simulink model "generic_HELP_ME_mu"  (R2025a)
settings: Solver=ode45  StartTime=0.0  StopTime=12  RelTol=1e-3  EnableMultiTasking=on
values from neighbouring files (symbols this model uses):
  Battery =     [Battery_A123_Pack_204s2p_Final.mat]
  cs_tyre = 2.0e5    (= 200000)    [mu_estimator_parameters.m]
  dOCV_dSoC = gradient(OCV, SoC_bp)    [SoCOcv.m]
  dR0 = gradient(R0, SoC_L)    [SoCOcv.m]
  eps_vx = 0.5    [mu_estimator_parameters.m]
  fz_max = 6000    [mu_estimator_parameters.m]
  fz_min = 300    [mu_estimator_parameters.m]
  h_cg = 0.55    [mu_estimator_parameters.m]
  lf = 1.214    [mu_estimator_parameters.m]
  lr = 1.505    [mu_estimator_parameters.m]
  r0 = 0.344    [mu_estimator_parameters.m]
  re_max = 0.33    [mu_estimator_parameters.m]
  re_min = 0.28    [mu_estimator_parameters.m]
  SoC_bp = Table_SoCvsOCV.LUT.SoC_percent    [SoCOcv.m]
  SoC_L = Battery.SOC_LUT    [SoCOcv.m]
  Table_SoCvsOCV = load("SoC_to_Voltage_LUT_10000-GON.mat")    [SoCOcv.m]
  tw_f = 1.571    [mu_estimator_parameters.m]
  tw_r = 1.581    [mu_estimator_parameters.m]
undefined symbols (not defined in the file or in its folder): DiscIntNeverNeededParam, Init_SoC
libraries: CarMaker4SL x61, simulink x1
(part 4 of 4)

== matlab function generic_HELP_ME_mu/CarMaker/MATLAB Function28 ==
  data: mhat input; fz_fl output; ax_eff input; ay input; lf input; lr input; h_cg input; fz_fr output; fz_rl output; fz_rr output; tw_f input; tw_r input; fz_front_total output; fz_rear_total output
function [fz_fl, fz_fr, fz_rl, fz_rr, fz_front_total, fz_rear_total] = ...
    vertical_load_combined(mhat, ax_eff, ay, lf, lr, h_cg, tw_f, tw_r)

g = 9.81;
kf = 0.55;
kr = 0.45;
fz_min = 300;

L = lf + lr;

% Transfert longitudinal
fz_front_total = (mhat * g * lr - mhat * ax_eff * h_cg) / L;
fz_rear_total  = (mhat * g * lf + mhat * ax_eff * h_cg) / L;

% Transfert lateral
dfz_f_lat = (mhat * ay * h_cg / tw_f) * kf;
dfz_r_lat = (mhat * ay * h_cg / tw_r) * kr;

% Charges roue par roue
fz_fl = fz_front_total/2 + dfz_f_lat/2;
fz_fr = fz_front_total/2 - dfz_f_lat/2;

fz_rl = fz_rear_total/2 + dfz_r_lat/2;
fz_rr = fz_rear_total/2 - dfz_r_lat/2;

% Saturation mini
fz_fl = max(fz_fl, fz_min);
fz_fr = max(fz_fr, fz_min);
fz_rl = max(fz_rl, fz_min);
fz_rr = max(fz_rr, fz_min);

% Totaux recalcules
fz_front_total = fz_fl + fz_fr;
fz_rear_total  = fz_rl + fz_rr;

== matlab function generic_HELP_ME_mu/CarMaker/MATLAB Function29 ==
  data: fz_fl input; re_fl output; fz_fr input; fz_rl input; fz_rr input; re_fr output; re_rl output; re_rr output; r0 input; cs_tyre input; re_min input; re_max input
function [re_fl, re_fr, re_rl, re_rr] = ...
    effective_radius(fz_fl, fz_fr, fz_rl, fz_rr, r0, cs_tyre, re_min, re_max)

re_fl = r0 - (2/3) * (fz_fl / cs_tyre);
re_fr = r0 - (2/3) * (fz_fr / cs_tyre);
re_rl = r0 - (2/3) * (fz_rl / cs_tyre);
re_rr = r0 - (2/3) * (fz_rr / cs_tyre);

re_fl = min(max(re_fl, re_min), re_max);
re_fr = min(max(re_fr, re_min), re_max);
re_rl = min(max(re_rl, re_min), re_max);
re_rr = min(max(re_rr, re_min), re_max);

== matlab function generic_HELP_ME_mu/CarMaker/MATLAB Function30 ==
  data: vx input; slip_fl output; omega_fl input; omega_fr input; omega_rl input; slip_fr output; slip_rl output; slip_rr output; omega_rr input; re_fl input; re_fr input; re_rl input; re_rr input; eps_vx input
function [slip_fl, slip_fr, slip_rl, slip_rr] = ...
    slip_estimator(vx, omega_fl, omega_fr, omega_rl, omega_rr, ...
                        re_fl, re_fr, re_rl, re_rr, eps_vx)

if abs(vx) < eps_vx
    slip_fl = 0;
    slip_fr = 0;
    slip_rl = 0;
    slip_rr = 0;
else
    slip_fl = (vx - omega_fl * re_fl) / max(abs(vx), eps_vx);
    slip_fr = (vx - omega_fr * re_fr) / max(abs(vx), eps_vx);
    slip_rl = (vx - omega_rl * re_rl) / max(abs(vx), eps_vx);
    slip_rr = (vx - omega_rr * re_rr) / max(abs(vx), eps_vx);

    slip_fl = min(max(slip_fl, 0), 1);
    slip_fr = min(max(slip_fr, 0), 1);
    slip_rl = min(max(slip_rl, 0), 1);
    slip_rr = min(max(slip_rr, 0), 1);
end

== matlab function generic_HELP_ME_mu/CarMaker/EKF ==
  settings: updateMethod=DISCRETE
  data: I input; soc_hat output; UL_meas input; Uoc input; R0_est input; R0nom input; R1 input; C1 input; dUoc_dSoc input; reset input; u1_hat output; ul_hat output; innov output; K_out output; P_out output; Qcap_est input; Qnom input
function [soc_hat, u1_hat, ul_hat, innov, K_out, P_out] = ...
    soc_ekf_paper_1rc(I, UL_meas, Uoc, R0_est, R0nom, R1, C1, dUoc_dSoc, reset, Qcap_est,Qnom)

    persistent x_hat P initialized

    Dt   = 0.01;
    Qnom = 3.6*Qnom;
    Qcap_est = Qcap_est*3600;
    

    Rekf = 1e-1;

    if isempty(initialized) || reset
        x_hat = [0.8;
                 0.0];

        P = [1e-6, 0;
             0,    1e-6];

        initialized = true;
    end

    
    if Qcap_est > 0
        Q0 = Qcap_est;
    else
        Q0 = Qnom;
    end

    
    if R0_est > 1e-3
        R0 = R0_est;
    else
        R0 = R0nom;
    end

    tau1 = R1 * C1;
    a1 = exp(-Dt / tau1);

    A = [1,  0;
         0, a1];

    B = [-Dt / Q0;
         R1 * (1 - exp(-Dt / tau1))];

    sigma_I2 = 1e-1;
    Q_input  = (B * B.') * sigma_I2;

    Q_base = [1e-8, 0;
              0,    1e-8];

    Qekf = Q_base + Q_input;

    % (1) State prediction
    x_pred = A * x_hat + B * I;

    % (2) Covariance prediction
    P_pred = A * P * A.' + Qekf;

    % (3) Measurement Jacobian
    C = [dUoc_dSoc, -1];

    % (4) Predicted output
    ul_hat = Uoc - R0 * I - x_pred(2);

    % (5) Kalman gain
    S = C * P_pred * C.' + Rekf;
    K = (P_pred * C.') / S;

    % (6) State update
    innov = UL_meas - ul_hat;
    x_hat = x_pred + K * innov;

    % (7) Covariance update
    I2 = eye(2);
    P = (I2 - K * C) * P_pred;

    % Outputs
    soc_hat = x_hat(1);
    u1_hat  = x_hat(2);
    K_out   = K;
    P_out   = P;
end

== matlab function generic_HELP_ME_mu/CarMaker/RC network subsystem/MATLAB Function ==
  data: I input; y output; R1 input; C1 input; V1 input
function y = fcn(I,R1,C1,V1)

y = -V1/(R1*C1)+I/C1;

== matlab function generic_HELP_ME_mu/CarMaker/Mass Estimator ==
  settings: updateMethod=DISCRETE
  data: y input; phi input; lambda input; m_hat output; t input; ax input
function m_hat = mass_rls(y, phi, lambda, t, ax)
    persistent theta P initialized t_start est_active done
    if isempty(initialized)
        theta = 1/2200;
        P = 1e6;
        t_start = 0;
        est_active = false;
        done = false;
        initialized = true;
    end
    theta_min = 1/3000;
    theta_max = 1/1500;
   
    if ~done && ~est_active && abs(ax) > 0.5
        est_active = true;
        t_start = t;
    end
   
    if est_active
        if (t - t_start) <= 10
            eps = y - phi * theta;
            L = (P * phi) / (lambda + phi * P * phi);
            theta = theta + L * eps;
            P = (P * (1 - L * phi)) / lambda;
            if theta < theta_min
                theta = theta_min;
            elseif theta > theta_max
                theta = theta_max;
            end
        else
            est_active = false;
            done = true;
        end
    end
    m_hat = 1 / theta;
end

== matlab function generic_HELP_ME_mu/CarMaker/MATLAB Function2 ==
  data: ax input; y output; beta input
function y = compute_y(ax,beta) 
g=9.81; 
f=0.015; 
delta=1; 
y = delta*ax + g*f + g*sin(beta);
